simulink model "c5new"  (Simulink 9.3)
settings: Solver=VariableStepAuto  StartTime=0.0  StopTime=20  RelTol=1e-3
libraries: Solver_SF x1
settings Model: Creator=121884344  LastModifiedBy=121884344
settings DataIOCC: SaveFormat=Dataset  SignalLoggingSaveFormat=Dataset  ReturnWorkspaceOutputs=on
settings OptimizationCC: LifeSpan=auto
settings DebuggingCC: UnderspecifiedInitializationDetection=Simplified  MergeDetectMultiDrivingBlocksExec=error  FcnCallInpInsideContextMsg=error  SFUnexpectedBacktrackingDiag=error  SFNoUnconditionalDefaultTransitionDiag=error  SFExecutionAtInitializationDiag=warning  ArithmeticOperatorsInVariantConditions=error
settings HardwareCC: ProdBitPerPointer=64  ProdBitPerSizeT=64  ProdBitPerPtrDiffT=64  ProdLargestAtomicFloat=Float  ProdIntDivRoundTo=Zero  ProdEndianess=LittleEndian  ProdWordSize=64  ProdHWDeviceType=Intel->x86-64 (Windows64)
settings ModelReferenceCC: PropagateSignalLabelsOutOfModel=on
settings SFSimCC: SimUseLocalCustomCode=on
settings RTWCC: RTWUseLocalCustomCode=on
settings CodeAppCC: StateflowObjectComments=off
settings GRTTargetCC: TargetLangStandard=C99 (ISO)  CombineOutputUpdateFcns=on  GRTInterface=off
settings ConfigComp: CovMetricSettings=dwe  CovHtmlReporting=off  CovSaveCumulativeToWorkspaceVar=off  CovSaveSingleToWorkspaceVar=off  CovExternalEMLEnable=on

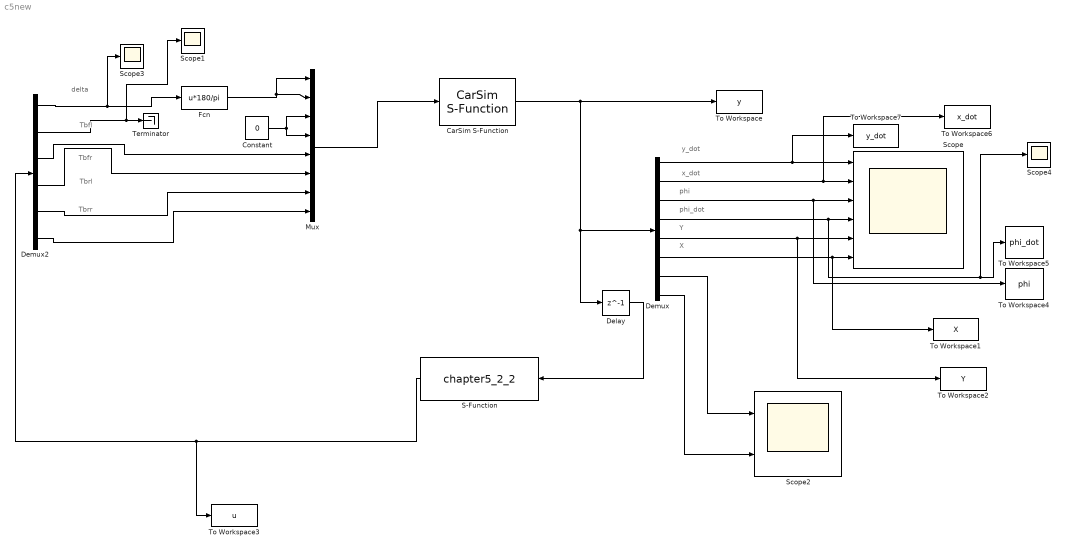
== system c5new ==
  note: Tbrr
  note: Tbrl
  note: Tbfr
  note: Tbfl
  note: X
  note: Y
  note: phi_dot
  note: phi
  note: x_dot
  note: y_dot
  note: delta
  CarSim S-Function : Solver_SF/CarSim S-Function  Priority=1  VehicleCode=i_i  SIMFILE=simfile
  Constant : Constant  Value=0
  Delay : Delay  DelayLength=1  InitialCondition=0
  Demux : Demux  Outputs=8
  Demux2 : Demux  Outputs=6
  Fcn : Fcn  Expr=u*180/pi
  Mux : Mux  Inputs=8
  S-Function : S-Function  FunctionName=chapter5_2_2  SFunctionDeploymentMode=off  EnableBusSupport=off
  Scope : Scope  NumInputPorts=6
  Scope1 : Scope
  Scope2 : Scope  NumInputPorts=2
  Scope3 : Scope
  Scope4 : Scope
  Terminator : Terminator
  To Workspace : ToWorkspace  VariableName=y  SaveFormat=Timeseries  SampleTime=-1
  To Workspace1 : ToWorkspace  VariableName=X  SaveFormat=Timeseries  SampleTime=-1
  To Workspace2 : ToWorkspace  VariableName=Y  SaveFormat=Timeseries  SampleTime=-1
  To Workspace3 : ToWorkspace  VariableName=u  SaveFormat=Timeseries  SampleTime=-1
  To Workspace4 : ToWorkspace  VariableName=phi  SampleTime=-1
      settings: Save2DSignal=2-D array (concatenate along first dimension)
  To Workspace5 : ToWorkspace  VariableName=phi_dot  SampleTime=-1
      settings: Save2DSignal=2-D array (concatenate along first dimension)
  To Workspace6 : ToWorkspace  VariableName=x_dot  SaveFormat=Timeseries  SampleTime=-1
  To Workspace7 : ToWorkspace  VariableName=y_dot  SaveFormat=Timeseries  SampleTime=-1
  wires:
  Fcn/1 -> Mux/1, Mux/2
  Constant/1 -> Mux/4, Mux/3
  Mux/1 -> CarSim S-Function/1
  CarSim S-Function/1 -> Delay/1, Demux/1, To Workspace/1
  Demux/1 -> To Workspace7/1, Scope/1
  Demux/2 -> To Workspace6/1, Scope/2
  Demux/3 -> To Workspace4/1, Scope/3
  Demux/4 -> Scope4/1, To Workspace5/1, Scope/4
  Demux/5 -> To Workspace2/1, Scope/5
  Demux/6 -> To Workspace1/1, Scope/6
  Delay/1 -> S-Function/1
  Demux/7 -> Scope2/1
  Demux/8 -> Scope2/2
  S-Function/1 -> Demux2/1, To Workspace3/1
  Demux2/1 -> Scope3/1, Fcn/1
  Demux2/3 -> Mux/5
  Demux2/4 -> Mux/6
  Demux2/5 -> Mux/7
  Demux2/6 -> Mux/8
  Demux2/2 -> Scope1/1, Terminator/1
